simulink model "simulatore_secondo_esercizio"  (R2024a)
settings: Solver=VariableStepAuto  StartTime=0.0  StopTime=10  RelTol=1e-3
undefined symbols (not defined in the file): den1, den2, den3, denc, denp, num1, num2, num3, numc, nump, Ts
settings Model: Creator=francesco  LastModifiedBy=rober
settings DebuggingCC: UnconnectedInputMsg=warning  UnconnectedOutputMsg=warning  UnconnectedLineMsg=warning
settings ModelReferenceCC: EnableRefExpFcnMdlSchedulingChecks=on
settings RTWCC: GPUComputeCapability=3.5  DLArmComputeVersion=19.05

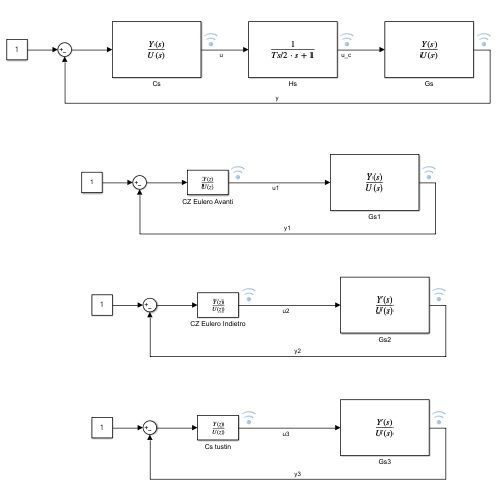
[thumbnail: Simulink's stored preview of the top-level diagram]
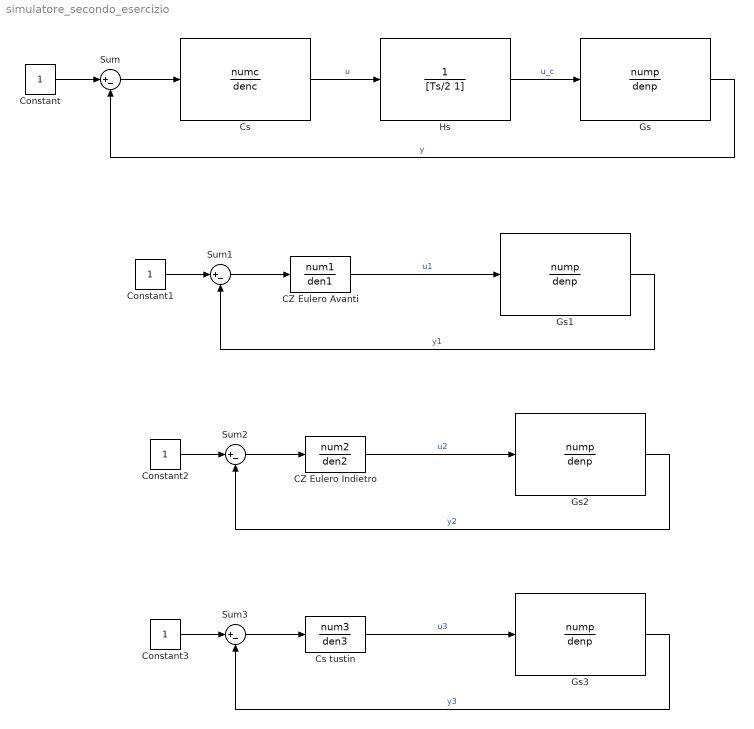
== system simulatore_secondo_esercizio ==
  CZ Eulero Avanti : DiscreteTransferFcn  Numerator=num1  Denominator=den1  SampleTime=Ts
  CZ Eulero Indietro : DiscreteTransferFcn  Numerator=num2  Denominator=den2  SampleTime=Ts
  Constant{,1..3} (4 alike) : Constant
  Cs : TransferFcn  Numerator=numc  Denominator=denc
  Cs tustin : DiscreteTransferFcn  Numerator=num3  Denominator=den3  SampleTime=Ts
  Gs{,1..3} (4 alike) : TransferFcn  Numerator=nump  Denominator=denp
  Hs : TransferFcn  Numerator=1  Denominator=[Ts/2 1]
  Sum{,1..3} (4 alike) : Sum  Inputs=|+-
  wires:
  Sum/1 -> Cs/1
  Cs/1 -> Hs/1  "u"
  Constant/1 -> Sum/1
  Gs/1 -> Sum/2  "y"
  Gs1/1 -> Sum1/2  "y1"
  Constant1/1 -> Sum1/1
  CZ Eulero Avanti/1 -> Gs1/1  "u1"
  Sum1/1 -> CZ Eulero Avanti/1
  Sum2/1 -> CZ Eulero Indietro/1
  CZ Eulero Indietro/1 -> Gs2/1  "u2"
  Constant2/1 -> Sum2/1
  Gs2/1 -> Sum2/2  "y2"
  Gs3/1 -> Sum3/2  "y3"
  Constant3/1 -> Sum3/1
  Cs tustin/1 -> Gs3/1  "u3"
  Sum3/1 -> Cs tustin/1
  Hs/1 -> Gs/1  "u_c"
